simulink model "PID_basic"  (R2016a)
settings: Solver=VariableStepAuto  StartTime=0.0  StopTime=20  RelTol=1e-3
libraries: simulink x1
settings Model: Creator=Administrator  LastModifiedBy=Administrator

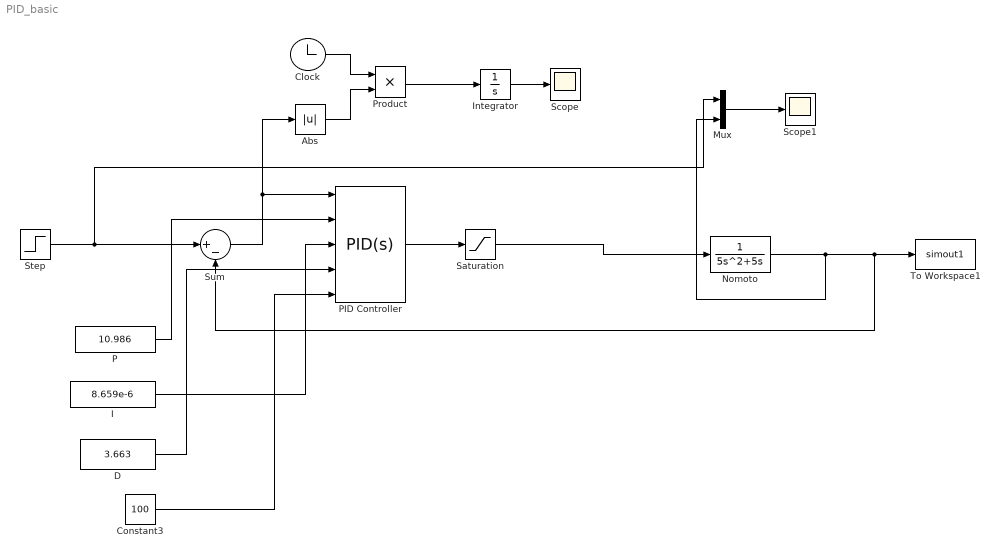
== system PID_basic ==
  Abs : Abs
  Clock : Clock
  Constant3 : Constant  Value=100
  D : Constant  Value=3.663
  I : Constant  Value=8.659e-6
  Integrator : Integrator
  Mux : Mux  Inputs=2
  Nomoto : TransferFcn  Denominator=[5 5 0]
  P : Constant  Value=10.986
  PID Controller : simulink/Continuous/PID Controller  Controller=PID  TimeDomain=Continuous-time  SampleTime=-1  IntegratorMethod=Forward Euler  FilterMethod=Forward Euler  Form=Parallel  UseFilter=on  ControllerParametersSource=external  P=1  I=1  D=0  N=100  InitialConditionSource=internal  InitialConditionForIntegrator=0  InitialConditionForFilter=0  ExternalReset=none  IgnoreLimit=on  ZeroCross=off  LimitOutput=off  UpperSaturationLimit=inf  LowerSaturationLimit=-inf  LinearizeAsGain=on  AntiWindupMode=none  Kb=1  TrackingMode=off  Kt=1  PParamMin=[]  PParamMax=[]  IParamMin=[]  IParamMax=[]  DParamMin=[]  DParamMax=[]  NParamMin=[]  NParamMax=[]  KbParamMin=[]  KbParamMax=[]  KtParamMin=[]  KtParamMax=[]  POutMin=[]  POutMax=[]  IOutMin=[]  IOutMax=[]  DOutMin=[]  DOutMax=[]  NOutMin=[]  NOutMax=[]  KbOutMin=[]  KbOutMax=[]  KtOutMin=[]  KtOutMax=[]  IntegratorOutMin=[]  IntegratorOutMax=[]  FilterOutMin=[]  FilterOutMax=[]  SumOutMin=[]  SumOutMax=[]  SumI1OutMin=[]  SumI1OutMax=[]  SumI2OutMin=[]  SumI2OutMax=[]  SumI3OutMin=[]  SumI3OutMax=[]  SumDOutMin=[]  SumDOutMax=[]  SaturationOutMin=[]  SaturationOutMax=[]  IntegratorContinuousStateAttributes=''  IntegratorStateMustResolveToSignalObject=off  IntegratorRTWStateStorageClass=Auto  FilterContinuousStateAttributes=''  FilterStateMustResolveToSignalObject=off  FilterRTWStateStorageClass=Auto  DifferentiatorICPrevScaledInput=0  DifferentiatorOutMin=[]  DifferentiatorOutMax=[]
  Product : Product
  Saturation : Saturate  UpperLimit=2  LowerLimit=-2
  Scope : Scope
  Scope1 : Scope
  Step : Step  Time=10  SampleTime=0
  Sum : Sum  Inputs=|+-
  To Workspace1 : ToWorkspace  VariableName=simout1  SampleTime=-1
  wires:
  Step/1 -> Mux/1, Sum/1
  Nomoto/1 -> Mux/2, To Workspace1/1, Sum/2
  Clock/1 -> Product/1
  Sum/1 -> Abs/1, PID Controller/1
  Product/1 -> Integrator/1
  Saturation/1 -> Nomoto/1
  Abs/1 -> Product/2
  PID Controller/1 -> Saturation/1
  Constant3/1 -> PID Controller/5
  D/1 -> PID Controller/4
  I/1 -> PID Controller/3
  P/1 -> PID Controller/2
  Integrator/1 -> Scope/1
  Mux/1 -> Scope1/1
